simulink model "Gain_design"  (R2016a)
settings: Solver=VariableStepAuto  StartTime=0.0  StopTime=10.0  RelTol=1e-3
settings Model: Creator=malikeh  LastModifiedBy=malikeh

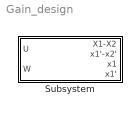
== system Gain_design ==
  Subsystem : Subsystem

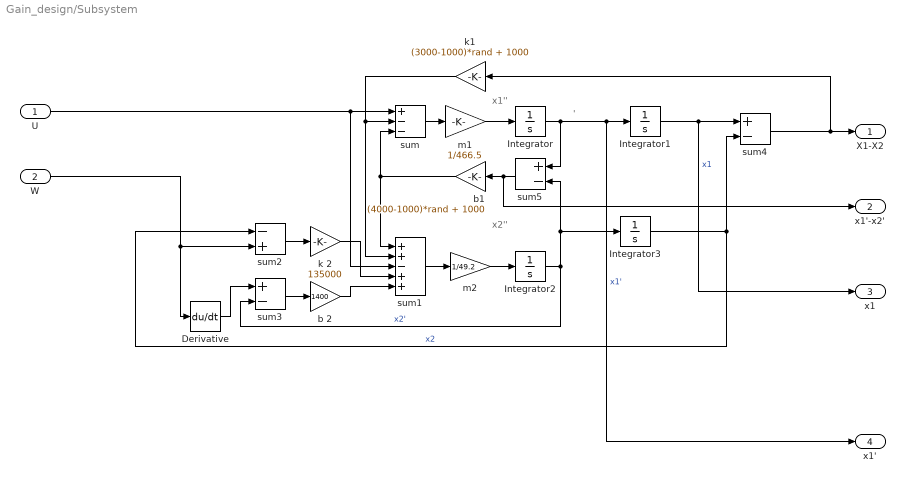
== system Gain_design/Subsystem ==
  note: x1''
  note: '
  note: x2''
  U : Inport
  W : Inport  Port=2
  " b1" : Gain  Gain=(4000-1000)*rand + 1000  SaturateOnIntegerOverflow=on  OutDataTypeStr=Inherit: Same as input  ParamDataTypeStr=Inherit: Same as input
  " k1" : Gain  Gain=(3000-1000)*rand + 1000  SaturateOnIntegerOverflow=on  OutDataTypeStr=Inherit: Same as input  ParamDataTypeStr=Inherit: Same as input
  Derivative : Derivative
  Integrator{,1..3} (4 alike) : Integrator
  b 2 : Gain  Gain=1400  SaturateOnIntegerOverflow=on  OutDataTypeStr=Inherit: Same as input  ParamDataTypeStr=Inherit: Same as input
  k 2 : Gain  Gain=135000  SaturateOnIntegerOverflow=on  OutDataTypeStr=Inherit: Same as input  ParamDataTypeStr=Inherit: Same as input
  m1 : Gain  Gain=1/466.5  SaturateOnIntegerOverflow=on  OutDataTypeStr=Inherit: Same as input  ParamDataTypeStr=Inherit: Same as input
  m2 : Gain  Gain=1/49.2  SaturateOnIntegerOverflow=on  OutDataTypeStr=Inherit: Same as input  ParamDataTypeStr=Inherit: Same as input
  sum : Sum  Inputs=+--  SaturateOnIntegerOverflow=on  InputSameDT=on  OutDataTypeStr=Inherit: Same as first input
  sum1 : Sum  Inputs=++-++  SaturateOnIntegerOverflow=on  InputSameDT=on  OutDataTypeStr=Inherit: Same as first input
  sum2 : Sum  Inputs=-+  SaturateOnIntegerOverflow=on  InputSameDT=on  OutDataTypeStr=Inherit: Same as first input
  sum3 : Sum  Inputs=+-  SaturateOnIntegerOverflow=on  InputSameDT=on  OutDataTypeStr=Inherit: Same as first input
  sum4 : Sum  Inputs=+-  SaturateOnIntegerOverflow=on  InputSameDT=on  OutDataTypeStr=Inherit: Same as first input
  sum5 : Sum  Inputs=+-  SaturateOnIntegerOverflow=on  InputSameDT=on  OutDataTypeStr=Inherit: Same as first input
  X1-X2 : Outport
  x1'-x2' : Outport  Port=2
  x1 : Outport  Port=3
  x1' : Outport  Port=4
  wires:
  m2/1 -> Integrator2/1
  sum1/1 -> m2/1
  Integrator2/1 -> sum5/2, Integrator3/1, sum3/2  "x2'"
  sum5/1 -> x1'-x2'/1, " b1"/1
  " b1"/1 -> sum1/1, sum/3
  m1/1 -> Integrator/1
  sum/1 -> m1/1
  Integrator1/1 -> x1/1, sum4/1  "x1"
  Integrator/1 -> x1'/1, Integrator1/1, sum5/1  "x1'"
  Integrator3/1 -> sum4/2, sum2/1  "x2"
  sum4/1 -> X1-X2/1, " k1"/1
  " k1"/1 -> sum/2, sum1/2
  b 2/1 -> sum1/5
  k 2/1 -> sum1/4
  sum2/1 -> k 2/1
  sum3/1 -> b 2/1
  U/1 -> sum/1, sum1/3
  Derivative/1 -> sum3/1
  W/1 -> Derivative/1, sum2/2
